simulink model "soc_range_doppler_fpga"  (R2025b)
settings: Solver=FixedStepDiscrete  StartTime=0.0  StopTime=inf  FixedStep=1/FPGAClkRate  RelTol=1e-3
values from neighbouring files (symbols this model uses):
  FPGAClkRate = Fs / SamplesPerClockCycle    (= 125000000)    [fmcw_run_test.m]    (also in soc_fmcw_init.m = 200000000)
  pulsePeriodSamples = ChirpSamples + 50    (= 1074)    [soc_range_doppler_system_param_init.m]    (also in soc_range_doppler_system_param_init_PDR_backup.m = 1952)
  pulseWidthSamples = 32    [soc_range_doppler_system_param_init.m]    (also in soc_range_doppler_system_param_init_PDR_backup.m)
  RngDimLen = ChirpSamples    (= 1024)    [soc_fmcw_init.m]    (also in soc_range_doppler_system_param_init.m; soc_range_doppler_system_param_init_PDR_backup.m)
  RxActiveSamples = ChirpSamples    (= 1024)    [soc_range_doppler_system_param_init.m]    (also in soc_range_doppler_system_param_init_PDR_backup.m)
  SamplesPerClockCycle = 2    [fmcw_run_test.m]    (also in soc_fmcw_init.m)
  TsFPGA = 1 / FPGAClkRate    (= 5e-09)    [soc_fmcw_init.m]
  txSignal = exp(1j * chirpPhase_short)    [soc_range_doppler_system_param_init.m]    (also in soc_range_doppler_system_param_init_PDR_backup.m = txSignalFullPeriod(1:pulseWidthSamples))
  VelDimLen = CPILength    (= 256)    [soc_fmcw_init.m]    (also in soc_range_doppler_system_param_init.m = 64; soc_range_doppler_system_param_init_PDR_backup.m = 64)
undefined symbols (not defined in the file or in its folder): NumBits1, NumBits2, TargetEmulator_MaxDelayLength, TargetEmulator_NCO_out_wl, TargetEmulator_NumChannels
libraries: simulink x9, socmemlib x8, hdlsllib x7, hwlogicconnlib x3, dsphdlsigops2 x1
(part 1 of 2)
settings Model: DataTypeOverride=Off  ModifiedByFormat=The MathWorks, Inc.  Creator=The MathWorks, Inc.  LastModifiedBy=The MathWorks, Inc.
settings SolverCC: AlgebraicLoopSolver=TrustRegion
settings DataIOCC: LimitDataPoints=on  SaveFormat=Array  SaveOutput=off  SaveTime=off  ReturnWorkspaceOutputs=off
settings OptimizationCC: BlockReduction=off  ConditionallyExecuteInputs=off  DefaultParameterBehavior=Inlined  ReuseModelBlockBuffer=off  LifeSpan=inf
settings DebuggingCC: AlgebraicLoopMsg=error  SolverPrmCheckMsg=warning  InheritedTsInSrcMsg=none  SingleTaskRateTransMsg=error  IntegerOverflowMsg=none  ParameterPrecisionLossMsg=none  UnconnectedInputMsg=warning  UnconnectedOutputMsg=warning  UnconnectedLineMsg=warning  AllowSymbolicDim=off  SFUnexpectedBacktrackingDiag=warning  SFNoUnconditionalDefaultTransitionDiag=warning  SFExecutionAtInitializationDiag=none  IntegerSaturationMsg=none  ArithmeticOperatorsInVariantConditions=warning
settings HardwareCC: ProdBitPerPointer=32.0  ProdBitPerSizeT=32.0  ProdBitPerPtrDiffT=32.0  ProdLargestAtomicFloat=None  ProdIntDivRoundTo=Undefined  ProdEndianess=Unspecified  ProdWordSize=32.0  ProdHWDeviceType=ASIC/FPGA->ASIC/FPGA  TargetBitPerPointer=64.0  TargetBitPerSizeT=64.0  TargetBitPerPtrDiffT=64.0  TargetLongLongMode=on  TargetIntDivRoundTo=Zero  TargetEndianess=LittleEndian  TargetWordSize=64.0  TargetHWDeviceType=Custom Processor->MATLAB Host Computer  ProdEqTarget=off
settings ModelReferenceCC: EnableRefExpFcnMdlSchedulingChecks=on  ModelReferenceNumInstancesAllowed=Single  PropagateSignalLabelsOutOfModel=off
settings SFSimCC: SimUseLocalCustomCode=off  CustomCodeUndefinedFunction=UseInterfaceOnly
settings RTWCC: RTWUseLocalCustomCode=off  GPUComputeCapability=3.5  DLArmComputeVersion=19.05
settings CodeAppCC: StateflowObjectComments=on
settings GRTTargetCC: TargetLangStandard=C89/C90 (ANSI)  SubcomponentCodeInterfacePackaging=Nonreusable function
settings ConfigComp: CovMetricSettings=dw  CovSaveCumulativeToWorkspaceVar=on  CovSaveSingleToWorkspaceVar=on  CovExternalEMLEnable=off  CovSFcnEnable=off
settings SimscapeCC: SimscapeNormalizeSystem=off

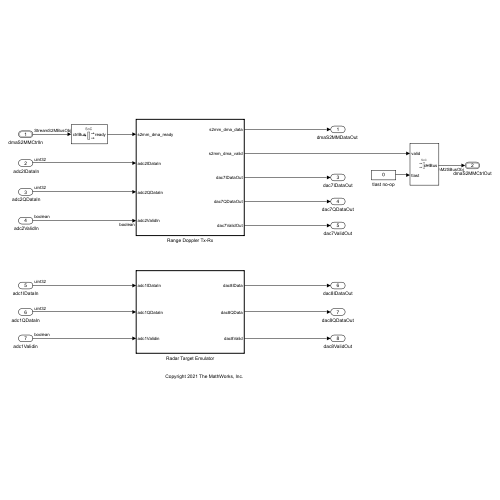
[thumbnail: Simulink's stored preview of the top-level diagram]
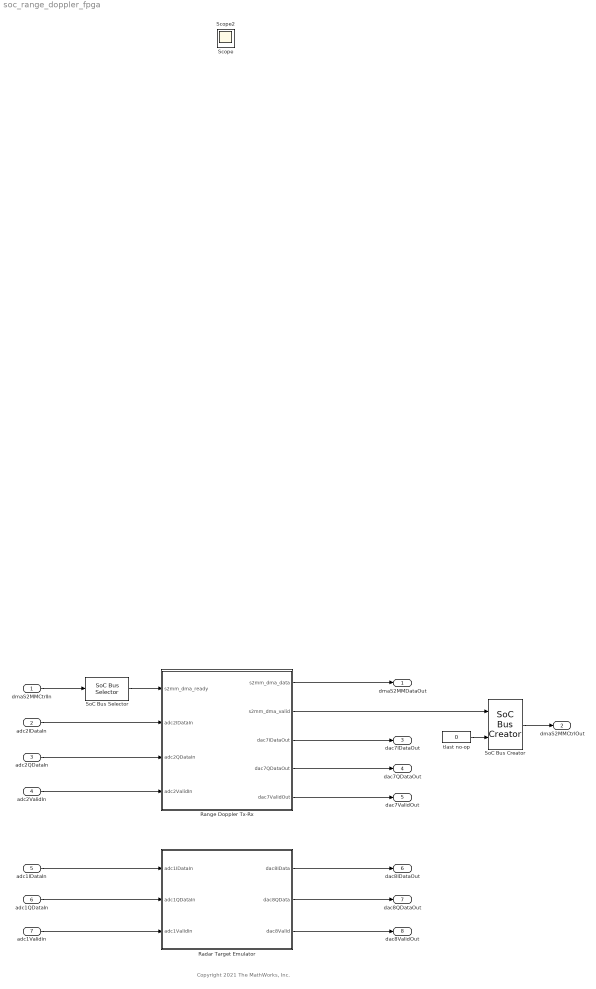
== system soc_range_doppler_fpga ==
  note: Copyright 2021 The MathWorks, Inc.
  dmaS2MMCtrlIn : Inport  OutDataTypeStr=Bus: StreamS2MBusObj  BusOutputAsStruct=on
  " adc2IDataIn" : Inport  Port=2  OutDataTypeStr=uint32  SampleTime=1/FPGAClkRate
  " adc2QDataIn" : Inport  Port=3  OutDataTypeStr=uint32  SampleTime=1/FPGAClkRate
  " adc2ValidIn" : Inport  Port=4  OutDataTypeStr=boolean  SampleTime=1/FPGAClkRate
  adc1IDataIn : Inport  Port=5  OutDataTypeStr=uint32
  adc1QDataIn : Inport  Port=6  OutDataTypeStr=uint32
  adc1Validin : Inport  Port=7  OutDataTypeStr=boolean
  Radar Target Emulator : Subsystem  TreatAsAtomicUnit=on
  Range Doppler Tx-Rx : Subsystem  TreatAsAtomicUnit=on
  SoC Bus Creator : hwlogicconnlib/SoC Bus Creator  Protocol=Data stream  ctrltype=Valid
  SoC Bus Selector : hwlogicconnlib/SoC Bus Selector  Protocol=Data stream  ctrltype=Ready
  tlast no-op : Constant  Value=0  OutDataTypeStr=boolean  SampleTime=-1
  "dmaS2MMDataOut " : Outport
  dmaS2MMCtrlOut : Outport  Port=2  OutDataTypeStr=Bus: StreamM2SBusObj  BusOutputAsStruct=on
  dac7IDataOut : Outport  Port=3
  dac7QDataOut : Outport  Port=4
  dac7ValidOut : Outport  Port=5
  dac8IDataOut : Outport  Port=6
  dac8QDataOut : Outport  Port=7
  dac8ValidOut : Outport  Port=8
  Scope : Scope
      settings: TimeSpan=1e-8*10  TimeUnits=Metric (based on Time Span)  ActiveDisplayYMinimum=-0.125  ActiveDisplayYMaximum=1.125
  Scope2 : Scope
      settings: ActiveDisplayYMinimum=-0.125  ActiveDisplayYMaximum=1.125
  wires:
  SoC Bus Creator/1 -> dmaS2MMCtrlOut/1
  tlast no-op/1 -> SoC Bus Creator/2
  Range Doppler Tx-Rx/2(s2mm_dma_valid) -> SoC Bus Creator/1
  SoC Bus Selector/1 -> Range Doppler Tx-Rx/1(s2mm_dma_ready)
  dmaS2MMCtrlIn/1 -> SoC Bus Selector/1
  Range Doppler Tx-Rx/1(s2mm_dma_data) -> "dmaS2MMDataOut "/1
  " adc2ValidIn"/1 -> Range Doppler Tx-Rx/4(adc2ValidIn)
  " adc2QDataIn"/1 -> Range Doppler Tx-Rx/3(adc2QDataIn)
  " adc2IDataIn"/1 -> Range Doppler Tx-Rx/2(adc2IDataIn)
  Radar Target Emulator/2(dac8QData) -> dac8QDataOut/1
  adc1IDataIn/1 -> Radar Target Emulator/1(adc1IDataIn)
  Radar Target Emulator/1(dac8IData) -> dac8IDataOut/1
  adc1Validin/1 -> Radar Target Emulator/3(adc1Validin)
  Radar Target Emulator/3(dac8Valid) -> dac8ValidOut/1
  adc1QDataIn/1 -> Radar Target Emulator/2(adc1QDataIn)
  Range Doppler Tx-Rx/3(dac7IDataOut) -> dac7IDataOut/1
  Range Doppler Tx-Rx/4(dac7QDataOut) -> dac7QDataOut/1
  Range Doppler Tx-Rx/5(dac7ValidOut) -> dac7ValidOut/1

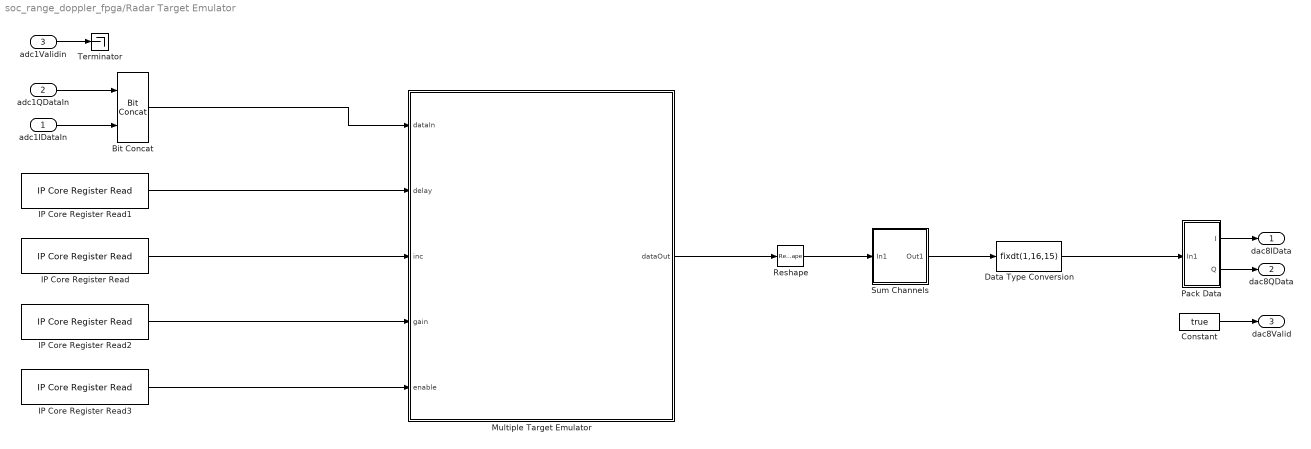
== system soc_range_doppler_fpga/Radar Target Emulator ==
  adc1IDataIn : Inport
  adc1QDataIn : Inport  Port=2
  adc1Validin : Inport  Port=3
  Bit Concat : hdlsllib/Logic and Bit Operations/Bit Concat  numInputs=2
  Constant : Constant  Value=true  SampleTime=-1
  Data Type Conversion : DataTypeConversion  OutDataTypeStr=fixdt(1,16,15)  SaturateOnIntegerOverflow=off  RndMeth=Floor
  IP Core Register Read : socmemlib/IP Core Register Read  RegisterName=Target_Emulator_Doppler_Inc  OutDataTypeStr=int32  OutputVectorSize=4  SampleTime=TsFPGA
  IP Core Register Read1 : socmemlib/IP Core Register Read  RegisterName=Target_Emulator_Range_Delay  OutDataTypeStr=uint32  OutputVectorSize=4  SampleTime=TsFPGA
  IP Core Register Read2 : socmemlib/IP Core Register Read  RegisterName=Target_Emulator_Gain  OutDataTypeStr=fixdt(1,18,17)  OutputVectorSize=4  SampleTime=TsFPGA
  IP Core Register Read3 : socmemlib/IP Core Register Read  RegisterName=Target_Emulator_Channel_Enable  OutDataTypeStr=boolean  OutputVectorSize=4  SampleTime=TsFPGA
  Multiple Target Emulator : Subsystem
  Pack Data : Subsystem
  Reshape : Reshape  OutputDimensionality=Customize  OutputDimensions=[SamplesPerClockCycle,TargetEmulator_NumChannels]
  Sum Channels : Subsystem
  Terminator : Terminator
  dac8IData : Outport
  dac8QData : Outport  Port=2
  dac8Valid : Outport  Port=3
  wires:
  adc1Validin/1 -> Terminator/1
  Constant/1 -> dac8Valid/1
  adc1IDataIn/1 -> Bit Concat/2
  adc1QDataIn/1 -> Bit Concat/1
  Pack Data/1(I) -> dac8IData/1
  Pack Data/2(Q) -> dac8QData/1
  Bit Concat/1 -> Multiple Target Emulator/1(dataIn)
  IP Core Register Read1/1 -> Multiple Target Emulator/2(delay)
  IP Core Register Read/1 -> Multiple Target Emulator/3(inc)
  IP Core Register Read2/1 -> Multiple Target Emulator/4(gain)
  Multiple Target Emulator/1(dataOut) -> Reshape/1
  Data Type Conversion/1 -> Pack Data/1(In1)
  IP Core Register Read3/1 -> Multiple Target Emulator/5(enable)
  Reshape/1 -> Sum Channels/1(In1)
  Sum Channels/1(Out1) -> Data Type Conversion/1

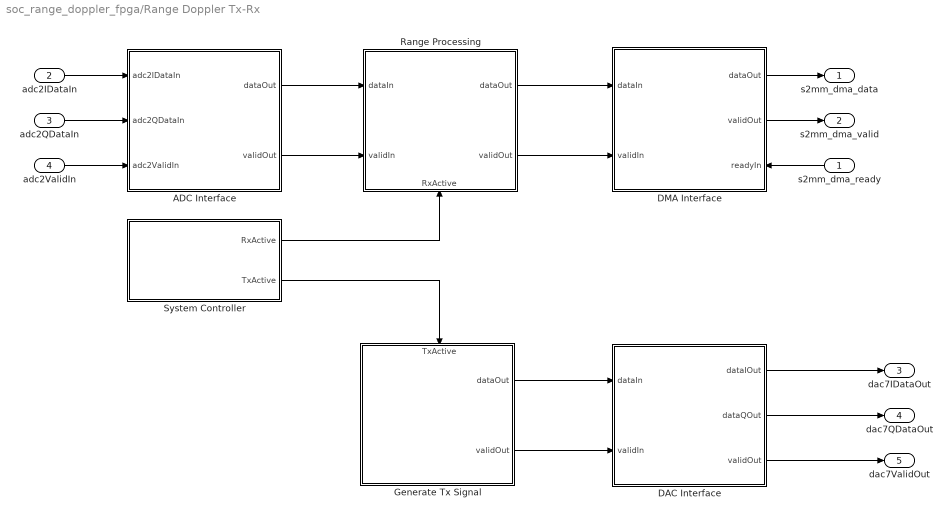
== system soc_range_doppler_fpga/Range Doppler Tx-Rx ==
  s2mm_dma_ready : Inport
  adc2IDataIn : Inport  Port=2  SampleTime=1/FPGAClkRate
  adc2QDataIn : Inport  Port=3  SampleTime=1/FPGAClkRate
  adc2ValidIn : Inport  Port=4  OutDataTypeStr=boolean  SampleTime=1/FPGAClkRate
  ADC Interface : Subsystem
  DAC Interface : Subsystem
  DMA Interface : Subsystem
      settings: PortSchema="{\"entries\":[{\"content\":{\"sides\":[{\"content\":{\"connectorIds\":[\"In1\",\"In2\"]},\"type\":\"ConnectorPlacement.EquallySpacedRectSide\",\"uuid\":\"5e6ee6ef-653d-4c22-91ec-0e4d08fe2bda\"},{\"content\":{\"connectorIds\":[\"Out1\",\"Out2\",\"In3\"],\"side\":\"RIGHT\"},\"type\":\"ConnectorPlacement.EquallySpacedRectSide\",\"uuid\":\"cc17ec3f-1a41-4b37-b05d-9322698b0460\"},{\"content\":{\"connectorIds\":[],\"side\":\"TOP\"},\"type\":\"ConnectorPlacement.EquallySpacedRectSide\",\"uuid\":\"ad44321b-ea67-4558-a5e3-5d4593ef958c\"},{\"content\":{\"connectorIds\":[],\"side\":\"HIDDEN\"},\"type\":\"ConnectorPlacement.EquallySpacedRectSide\",\"uuid\":\"4d1513b6-023e-4107-a61f-cebca5303f4a\"}]},\"type\":\"ConnectorPlacement.EquallySpacedConnector\",\"uuid\":\"368f7437-0e21-4f0c-b817-b9c98445f229\"}],\"packageUris\":[\"http://schema.mathworks.com/mf0/Connector/R2020b\"],\"version\":\"1.0\"}"
  Generate Tx Signal : Subsystem
      settings: PortSchema="{\"entries\":[{\"content\":{\"sides\":[{\"content\":{\"connectorIds\":[]},\"type\":\"ConnectorPlacement.EquallySpacedRectSide\",\"uuid\":\"7c0c8442-b2b4-479b-a8c5-9f379b7e9b02\"},{\"content\":{\"connectorIds\":[\"Out1\",\"Out2\"],\"side\":\"RIGHT\"},\"type\":\"ConnectorPlacement.EquallySpacedRectSide\",\"uuid\":\"78e009c0-26e1-4601-bc88-d3b747828f60\"},{\"content\":{\"connectorIds\":[\"In1\"],\"side\":\"TOP\"},\"type\":\"ConnectorPlacement.EquallySpacedRectSide\",\"uuid\":\"f420d1c4-59cf-4bc3-a158-4cd82eb58765\"},{\"content\":{\"connectorIds\":[],\"side\":\"BOTTOM\"},\"type\":\"ConnectorPlacement.EquallySpacedRectSide\",\"uuid\":\"c7f1fd46-69ec-4218-a957-5990432ef52d\"},{\"content\":{\"connectorIds\":[],\"side\":\"HIDDEN\"},\"type\":\"ConnectorPlacement.EquallySpacedRectSide\",\"uuid\":\"a6a12a6f-fd1c-4a75-bd3d-72d2093a42d1\"}]},\"type\":\"ConnectorPlacement.EquallySpacedConnector\",\"uuid\":\"fef31356-b6d9-440d-aa7f-68d9fbecd58b\"}],\"packageUris\":[\"http://schema.mathworks.com/mf0/Connector/R2020b\"],\"version\":\"1.0\"}"
  Range Processing : Subsystem
      settings: PortSchema="{\"entries\":[{\"content\":{\"sides\":[{\"content\":{\"connectorIds\":[\"In1\",\"In2\"]},\"type\":\"ConnectorPlacement.EquallySpacedRectSide\",\"uuid\":\"39bc8e28-b2f1-4549-a29c-f4f4cd813fa8\"},{\"content\":{\"connectorIds\":[\"Out1\",\"Out2\"],\"side\":\"RIGHT\"},\"type\":\"ConnectorPlacement.EquallySpacedRectSide\",\"uuid\":\"b450daac-133f-42c0-b4eb-be8f21a05aa1\"},{\"content\":{\"connectorIds\":[],\"side\":\"TOP\"},\"type\":\"ConnectorPlacement.EquallySpacedRectSide\",\"uuid\":\"67fab3c9-6d2a-4d44-89b3-69577d01f951\"},{\"content\":{\"connectorIds\":[\"In3\"],\"side\":\"BOTTOM\"},\"type\":\"ConnectorPlacement.EquallySpacedRectSide\",\"uuid\":\"f598741e-2794-4676-b4d9-8ec658bb222d\"},{\"content\":{\"connectorIds\":[],\"side\":\"HIDDEN\"},\"type\":\"ConnectorPlacement.EquallySpacedRectSide\",\"uuid\":\"bbc24f9c-adbc-4398-b2a6-1edaf7ae5a6a\"}]},\"type\":\"ConnectorPlacement.EquallySpacedConnector\",\"uuid\":\"0f1d461d-e89e-4ae5-bc4e-aa440f4196de\"}],\"packageUris\":[\"http://schema.mathworks.com/mf0/Connector/R2020b\"],\"version\":\"1.0\"}"
  System Controller : Subsystem
  s2mm_dma_data : Outport
  s2mm_dma_valid : Outport  Port=2
  dac7IDataOut : Outport  Port=3
  dac7QDataOut : Outport  Port=4
  dac7ValidOut : Outport  Port=5
  wires:
  DMA Interface/1(dataOut) -> s2mm_dma_data/1
  s2mm_dma_ready/1 -> DMA Interface/3(readyIn)
  DMA Interface/2(validOut) -> s2mm_dma_valid/1
  DAC Interface/1(dataIOut) -> dac7IDataOut/1
  DAC Interface/2(dataQOut) -> dac7QDataOut/1
  DAC Interface/3(validOut) -> dac7ValidOut/1
  System Controller/2(TxActive) -> Generate Tx Signal/1(TxActive)
  Range Processing/1(dataOut) -> DMA Interface/1(dataIn)
  System Controller/1(RxActive) -> Range Processing/3(RxActive)
  Generate Tx Signal/1(dataOut) -> DAC Interface/1(dataIn)
  Generate Tx Signal/2(validOut) -> DAC Interface/2(validIn)
  Range Processing/2(validOut) -> DMA Interface/2(validIn)
  ADC Interface/1(dataOut) -> Range Processing/1(dataIn)
  ADC Interface/2(validOut) -> Range Processing/2(validIn)
  adc2IDataIn/1 -> ADC Interface/1(adc2IDataIn)
  adc2QDataIn/1 -> ADC Interface/2(adc2QDataIn)
  adc2ValidIn/1 -> ADC Interface/3(adc2ValidIn)

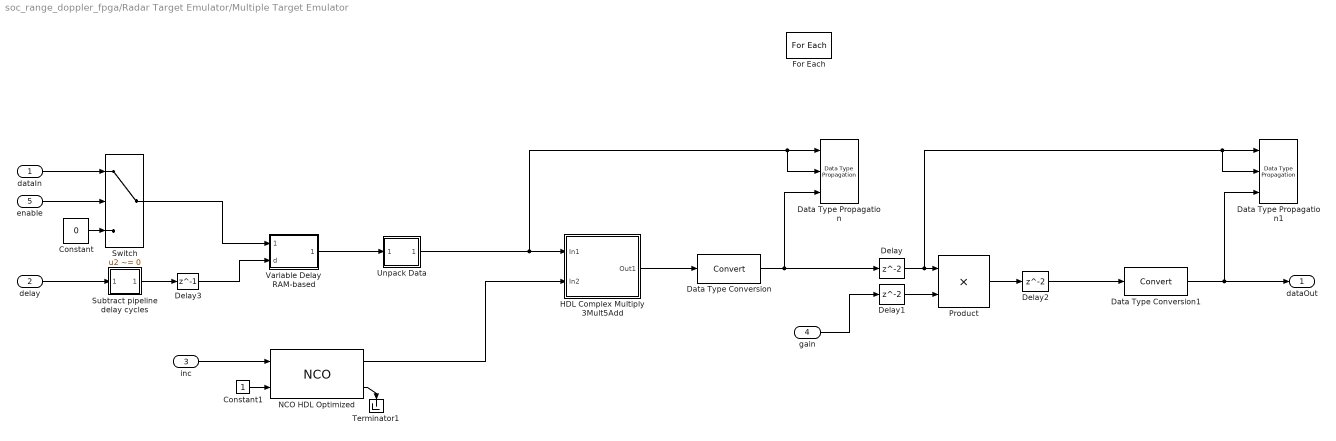
== system soc_range_doppler_fpga/Radar Target Emulator/Multiple Target Emulator ==
  dataIn : Inport
  delay : Inport  Port=2  Partition=on  PartitionDimension=1  PartitionWidth=1  PartitionOffset=0
  inc : Inport  Port=3  Partition=on  PartitionDimension=1  PartitionWidth=1  PartitionOffset=0
  gain : Inport  Port=4  Partition=on  PartitionDimension=1  PartitionWidth=1  PartitionOffset=0
  enable : Inport  Port=5  Partition=on  PartitionDimension=1  PartitionWidth=1  PartitionOffset=0
  Constant : Constant  Value=0  OutDataTypeStr=Inherit: Inherit via back propagation  SampleTime=-1
  Constant1 : Constant  OutDataTypeStr=boolean  SampleTime=-1
  Data Type Propagation : simulink/Signal Attributes/Data Type Propagation  PropDataTypeMode=Specify via dialog  PropDataType=fixdt(1, 24)  IfRefDouble=double  IfRefSingle=single  IsSigned=IsSigned1 or IsSigned2  NumBitsBase=max([NumBits1 NumBits2])  NumBitsMult=1  NumBitsAdd=0  NumBitsAllowFinal=1:24  PropScaling=2^-10  ValuesUsedBestPrec=[5 -7]  SlopeBase=PosRange1  SlopeMult=1  SlopeAdd=0  BiasBase=Bias1  BiasMult=1  BiasAdd=0
  Data Type Propagation1 : simulink/Signal Attributes/Data Type Propagation  PropDataTypeMode=Specify via dialog  PropDataType=fixdt(1, 16)  IfRefDouble=double  IfRefSingle=single  IsSigned=IsSigned1 or IsSigned2  NumBitsBase=max([NumBits1 NumBits2])  NumBitsMult=1  NumBitsAdd=0  NumBitsAllowFinal=1:24  PropScaling=2^-10  ValuesUsedBestPrec=[5 -7]  SlopeBase=PosRange1  SlopeMult=1  SlopeAdd=0  BiasBase=Bias1  BiasMult=1  BiasAdd=0
  Data Type Conversion : DataTypeConversion  SaturateOnIntegerOverflow=off  RndMeth=Floor
  Data Type Conversion1 : DataTypeConversion  SaturateOnIntegerOverflow=off  RndMeth=Floor
  Delay : Delay
  Delay1 : Delay
  Delay2 : Delay
  Delay3 : Delay  DelayLength=1
  For Each : ForEach  DisableCoverage=on
  HDL Complex Multiply 3Mult5Add : Subsystem  mask(HDL Complex Multiplier (3 Multiply, 5 Add)){D1=2, D2=1, D3=1, D4=1, D5=1}
      mask help:
      | Xilinx devices:
      | - Set D1 = 1 or 2 to trade off speed & FF resources
      | - Set D2-D5 = 1 to fully leverage DSP48 pipelines
      | - Use sync reset
      |
      | Intel FPGAs:
      | - Set D1 = 1 or 2 depending on device family
      | - Set D5 = 1; D2, D3, D4 = 0
      | - Use async reset
      mask init:
      | delay = D1+D2+D3+D4+D5;
  NCO HDL Optimized : dsphdlsigops2/NCO  PhaseIncrementSource=Input port  PhaseIncrement=100  PhaseOffsetSource=Property  PhaseOffset=0  DitherSource=Property  NumDitherBits=TargetEmulator_NCO_dither_wl  SamplesPerFrame=1  LUTCompress=on  ResetAction=off  Waveform=Complex exponential  PhasePort=off  SimulateUsing=Code generation  AccumulatorWL=TargetEmulator_NCO_accum_wl  PhaseQuantization=on  NumQuantizerAccumulatorBits=TargetEmulator_NCO_quantizer_wl  OutputDataType=Binary point scaling  OutputWL=TargetEmulator_NCO_out_wl  OutputFL=TargetEmulator_NCO_out_wl-1
  Product : Product
  Subtract pipeline delay cycles : Subsystem  mask{C=12 + nextpow2(TargetEmulator_NumChannels)}
      mask prompts: C "Constant"
      mask init:
      | dt = fixdt(1,nextpow2(C)+1,0);
      mask Display:
      | Cstr = get_param(gcb,'C');
      | 
      | fprintf('u-%s',Cstr);
  Switch : Switch  Criteria=u2 ~= 0  SaturateOnIntegerOverflow=off  InputSameDT=off
  Terminator1 : Terminator
  Unpack Data : Subsystem
  Variable Delay RAM-based : Subsystem  mask(RAM-based variable delay){MAX_DELAY=TargetEmulator_MaxDelayLength}
      mask prompts: MAX_DELAY "Maximum delay length:"
      mask TypeOptions MAX_DELAY: Variable Delay RAM Based/MAX_DELAY
      mask Display:
      | text(0.5,0.5,'z^{-d-1}','horizontalAlignment','center',...
      |     'verticalAlignment','middle','texmode','on');
      | 
      | port_label('input',1,'u');
      | port_label('input',2,'d');
  dataOut : Outport  ConcatenationDimension=1
  wires:
  NCO HDL Optimized/2 -> Terminator1/1
  Delay2/1 -> Data Type Conversion1/1
  Constant1/1 -> NCO HDL Optimized/2
  Delay3/1 -> Variable Delay RAM-based/2(d)
  Unpack Data/1(Out1) -> Data Type Propagation/2, Data Type Propagation/1, HDL Complex Multiply 3Mult5Add/1(In1)
  inc/1 -> NCO HDL Optimized/1
  Product/1 -> Delay2/1
  Variable Delay RAM-based/1(dataOut) -> Unpack Data/1(In1)
  Data Type Conversion/1 -> Data Type Propagation/3, Delay/1
  Subtract pipeline delay cycles/1(Out1) -> Delay3/1
  HDL Complex Multiply 3Mult5Add/1(Out1) -> Data Type Conversion/1
  NCO HDL Optimized/1 -> HDL Complex Multiply 3Mult5Add/2(In2)
  Data Type Conversion1/1 -> dataOut/1, Data Type Propagation1/3
  Delay/1 -> Data Type Propagation1/2, Data Type Propagation1/1, Product/1
  Delay1/1 -> Product/2
  delay/1 -> Subtract pipeline delay cycles/1(In1)
  gain/1 -> Delay1/1
  enable/1 -> Switch/2
  Switch/1 -> Variable Delay RAM-based/1(dataIn)
  dataIn/1 -> Switch/1
  Constant/1 -> Switch/3

== system soc_range_doppler_fpga/Radar Target Emulator/Pack Data ==
  In1 : Inport
  Complex to Real-Imag : ComplexToRealImag
  Pack Vector : Subsystem  mask(Pack Vector){}
      mask help:
      | Convert vector to packed word.
      |
      | The first vector element is placed in the LSB, and the last vector element is placed in the MSB.
      mask Display: fprintf('Pack\nVector');
  Pack Vector1 : Subsystem  mask(Pack Vector){}
      mask help:
      | Convert vector to packed word.
      |
      | The first vector element is placed in the LSB, and the last vector element is placed in the MSB.
      mask Display: fprintf('Pack\nVector');
  I : Outport
  Q : Outport  Port=2
  wires:
  In1/1 -> Complex to Real-Imag/1
  Complex to Real-Imag/1 -> Pack Vector/1(u)
  Complex to Real-Imag/2 -> Pack Vector1/1(u)
  Pack Vector/1(y) -> I/1
  Pack Vector1/1(y) -> Q/1

== system soc_range_doppler_fpga/Radar Target Emulator/Sum Channels ==
  In1 : Inport
  Delay : Delay  DelayLength=nextpow2(TargetEmulator_NumChannels)
  Sum of Elements : Sum  Inputs=+  CollapseMode=Specified dimension  CollapseDim=2
  Out1 : Outport
  wires:
  In1/1 -> Sum of Elements/1
  Sum of Elements/1 -> Delay/1
  Delay/1 -> Out1/1

== system soc_range_doppler_fpga/Range Doppler Tx-Rx/ADC Interface ==
  adc2IDataIn : Inport  SampleTime=1/FPGAClkRate
  adc2QDataIn : Inport  Port=2  SampleTime=1/FPGAClkRate
  adc2ValidIn : Inport  Port=3  OutDataTypeStr=boolean  SampleTime=1/FPGAClkRate
  Data Type Conversion2 : DataTypeConversion  OutDataTypeStr=inputDT  SaturateOnIntegerOverflow=off  RndMeth=Floor
  Real-Imag to Complex : RealImagToComplex
  Unpack Vector I : Subsystem  mask(Convert packed word to vector.){datatype=fixdt(1,16,15), VectorLength=SamplesPerClockCycle}
      mask prompts: datatype "Output datatype:"; VectorLength "Vector length:"
      mask help: Input word has the first vector element in the LSB and the last element in the MSB.
      mask init:
      | OutputWordLength = numerictype(datatype).WordLength;
      | 
      | Simulink.suppressDiagnostic(gcbh,...
      |  'SimulinkFixedPoint:util:Overflowoccurred');
      mask Display: fprintf('Unpack\nVector');
  Unpack Vector Q : Subsystem  mask(Convert packed word to vector.){datatype=fixdt(1,16,15), VectorLength=SamplesPerClockCycle}
      mask prompts: datatype "Output datatype:"; VectorLength "Vector length:"
      mask help: Input word has the first vector element in the LSB and the last element in the MSB.
      mask init:
      | OutputWordLength = numerictype(datatype).WordLength;
      | 
      | Simulink.suppressDiagnostic(gcbh,...
      |  'SimulinkFixedPoint:util:Overflowoccurred');
      mask Display: fprintf('Unpack\nVector');
  dataOut : Outport
  validOut : Outport  Port=2
  wires:
  adc2IDataIn/1 -> Unpack Vector I/1(In1)
  Real-Imag to Complex/1 -> Data Type Conversion2/1
  Unpack Vector Q/1(Out1) -> Real-Imag to Complex/2
  Unpack Vector I/1(Out1) -> Real-Imag to Complex/1
  Data Type Conversion2/1 -> dataOut/1
  adc2ValidIn/1 -> validOut/1
  adc2QDataIn/1 -> Unpack Vector Q/1(In1)

== system soc_range_doppler_fpga/Range Doppler Tx-Rx/DAC Interface ==
  dataIn : Inport
  validIn : Inport  Port=2
  Complex to Real-Imag : ComplexToRealImag
  Pack Vector I : Subsystem  mask(Pack Vector){}
      mask help:
      | Convert vector to packed word.
      |
      | The first vector element is placed in the LSB, and the last vector element is placed in the MSB.
      mask Display: fprintf('Pack\nVector');
  Pack Vector Q : Subsystem  mask(Pack Vector){}
      mask help:
      | Convert vector to packed word.
      |
      | The first vector element is placed in the LSB, and the last vector element is placed in the MSB.
      mask Display: fprintf('Pack\nVector');
  dataIOut : Outport
  dataQOut : Outport  Port=2
  validOut : Outport  Port=3
  wires:
  Complex to Real-Imag/1 -> Pack Vector I/1(u)
  Complex to Real-Imag/2 -> Pack Vector Q/1(u)
  Pack Vector I/1(y) -> dataIOut/1
  Pack Vector Q/1(y) -> dataQOut/1
  dataIn/1 -> Complex to Real-Imag/1
  validIn/1 -> validOut/1

== system soc_range_doppler_fpga/Range Doppler Tx-Rx/DMA Interface ==
  dataIn : Inport
  validIn : Inport  Port=2
  readyIn : Inport  Port=3
  Pack Complex Vector : Subsystem  mask(Pack Complex Vector){}
      mask help:
      | Convert complex vector to packed word.
      |
      | Real and imaginary components are interleaved, with real component starting in LSB position.
      |
      | The first vector element is placed in the LSB, and the last vector element is placed in the MSB.
      mask Display: fprintf('Pack\nComplex\nVector');
  Stream FIFO : hwlogicconnlib/Stream FIFO  FIFO_DEPTH=1024  AFULL_THRESH=1023
  Terminator : Terminator
  dataOut : Outport
  validOut : Outport  Port=2
  wires:
  dataIn/1 -> Pack Complex Vector/1(u)
  Stream FIFO/1 -> dataOut/1
  Stream FIFO/2 -> validOut/1
  readyIn/1 -> Stream FIFO/3
  Pack Complex Vector/1(y) -> Stream FIFO/1
  validIn/1 -> Stream FIFO/2
  Stream FIFO/3 -> Terminator/1

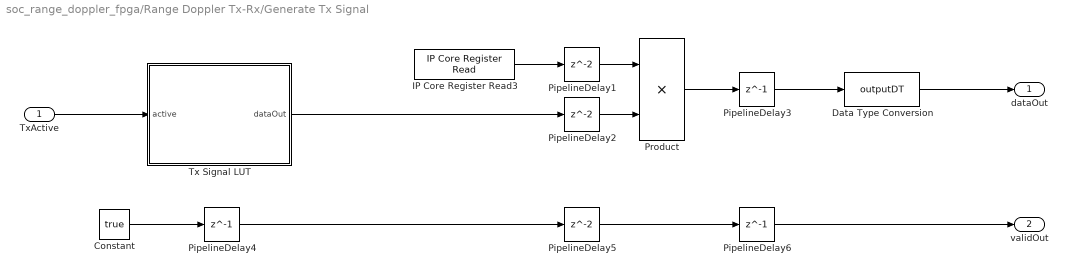
== system soc_range_doppler_fpga/Range Doppler Tx-Rx/Generate Tx Signal ==
  TxActive : Inport
  Constant : Constant  Value=true  SampleTime=-1
  Data Type Conversion : DataTypeConversion  OutDataTypeStr=outputDT  SaturateOnIntegerOverflow=off  RndMeth=Floor
  IP Core Register Read3 : socmemlib/IP Core Register Read  RegisterName=Tx_Gain  OutDataTypeStr=fixdt(1,18,16)  OutputVectorSize=1  SampleTime=TsFPGA
  PipelineDelay1 : Delay
  PipelineDelay2 : Delay
  PipelineDelay3 : Delay  DelayLength=1
  PipelineDelay4 : Delay  DelayLength=1
  PipelineDelay5 : Delay
  PipelineDelay6 : Delay  DelayLength=1
  Product : Product
  Tx Signal LUT : Subsystem
  dataOut : Outport
  validOut : Outport  Port=2
  wires:
  Product/1 -> PipelineDelay3/1
  PipelineDelay3/1 -> Data Type Conversion/1
  PipelineDelay2/1 -> Product/2
  PipelineDelay1/1 -> Product/1
  IP Core Register Read3/1 -> PipelineDelay1/1
  Tx Signal LUT/1(dataOut) -> PipelineDelay2/1
  TxActive/1 -> Tx Signal LUT/1(active)
  Data Type Conversion/1 -> dataOut/1
  Constant/1 -> PipelineDelay4/1
  PipelineDelay4/1 -> PipelineDelay5/1
  PipelineDelay5/1 -> PipelineDelay6/1
  PipelineDelay6/1 -> validOut/1

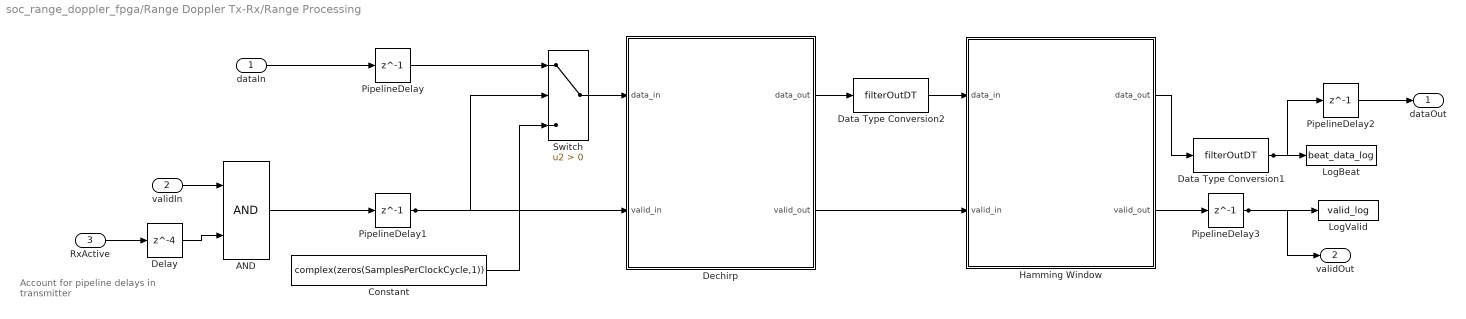
== system soc_range_doppler_fpga/Range Doppler Tx-Rx/Range Processing ==
  note: Account for pipeline
      | delays in transmitter
  dataIn : Inport
  validIn : Inport  Port=2
  RxActive : Inport  Port=3
  AND : Logic  IconShape=distinctive  AllPortsSameDT=off  OutDataTypeStr=boolean
  Constant : Constant  Value=complex(zeros(SamplesPerClockCycle,1))  OutDataTypeStr=inputDT  SampleTime=-1
  Data Type Conversion1 : DataTypeConversion  OutDataTypeStr=filterOutDT  SaturateOnIntegerOverflow=off  RndMeth=Floor
  Data Type Conversion2 : DataTypeConversion  OutDataTypeStr=filterOutDT  SaturateOnIntegerOverflow=off  RndMeth=Floor
  Dechirp : Subsystem
  Delay : Delay  DelayLength=4
  Hamming Window : Subsystem
  LogBeat : ToWorkspace  VariableName=beat_data_log  SaveFormat=Timeseries  SampleTime=-1
  LogValid : ToWorkspace  VariableName=valid_log  SaveFormat=Timeseries  SampleTime=-1
  PipelineDelay{,1..3} (4 alike) : Delay  DelayLength=1
  Switch : Switch  Criteria=u2 > Threshold  SaturateOnIntegerOverflow=off  InputSameDT=off
  dataOut : Outport
  validOut : Outport  Port=2
  wires:
  validIn/1 -> AND/1
  RxActive/1 -> Delay/1
  Constant/1 -> Switch/3
  PipelineDelay/1 -> Switch/1
  Delay/1 -> AND/2
  dataIn/1 -> PipelineDelay/1
  AND/1 -> PipelineDelay1/1
  PipelineDelay1/1 -> Dechirp/2(valid_in), Switch/2
  PipelineDelay2/1 -> dataOut/1
  Switch/1 -> Dechirp/1(data_in)
  Dechirp/1(data_out) -> Data Type Conversion2/1
  Dechirp/2(valid_out) -> Hamming Window/2(valid_in)
  Data Type Conversion2/1 -> Hamming Window/1(data_in)
  Hamming Window/1(data_out) -> Data Type Conversion1/1
  Hamming Window/2(valid_out) -> PipelineDelay3/1
  Data Type Conversion1/1 -> PipelineDelay2/1, LogBeat/1
  PipelineDelay3/1 -> validOut/1, LogValid/1

== system soc_range_doppler_fpga/Range Doppler Tx-Rx/System Controller ==
  IP Core Register Read : socmemlib/IP Core Register Read  RegisterName=CPI_Start  OutDataTypeStr=boolean  OutputVectorSize=1  SampleTime=TsFPGA
  IP Core Register Read1 : socmemlib/IP Core Register Read  RegisterName=CPI_Length  OutDataTypeStr=uint32  OutputVectorSize=1  SampleTime=TsFPGA
  IP Core Register Read2 : socmemlib/IP Core Register Read  RegisterName=Rx_Delay_Cycles  OutDataTypeStr=uint32  OutputVectorSize=1  SampleTime=TsFPGA
  System Controller Fcn : MATLAB Function  TreatAsAtomicUnit=on
  RxActive : Outport
  TxActive : Outport  Port=2
  wires:
  IP Core Register Read2/1 -> System Controller Fcn/3(rx_delay_cycles)
  IP Core Register Read1/1 -> System Controller Fcn/2(cpi_length)
  IP Core Register Read/1 -> System Controller Fcn/1(cpi_start)
  System Controller Fcn/1(tx_active) -> TxActive/1
  System Controller Fcn/2(rx_active) -> RxActive/1

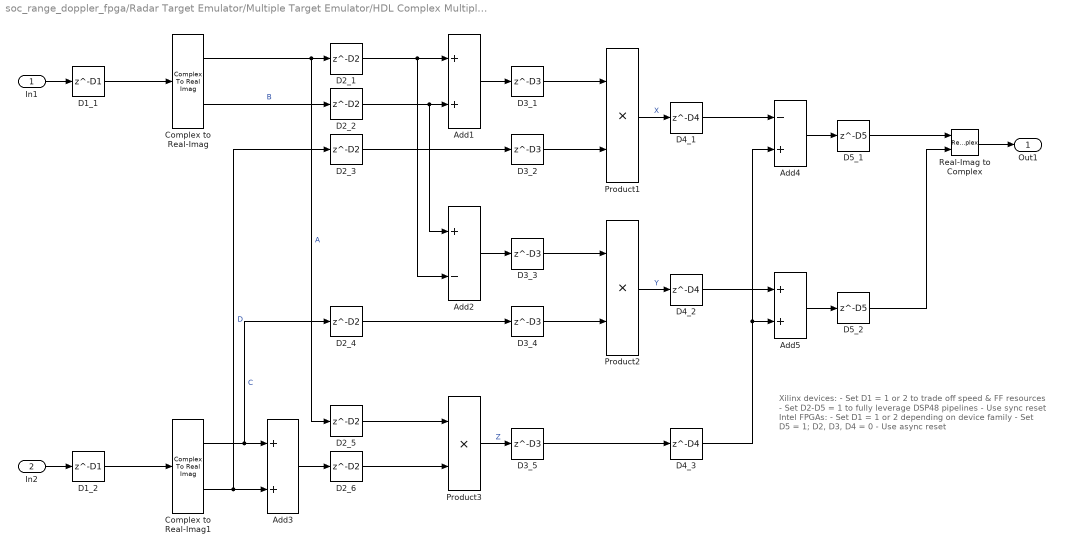
== system soc_range_doppler_fpga/Radar Target Emulator/Multiple Target Emulator/HDL Complex Multiply 3Mult5Add ==
  note: Xilinx devices:
      | - Set D1 = 1 or 2 to trade off speed & FF resources
      | - Set D2-D5 = 1 to fully leverage DSP48 pipelines
      | - Use sync reset
      |
      | Intel FPGAs:
      | - Set D1 = 1 or 2 depending on device family
      | - Set D5 = 1; D2, D3, D4 = 0
      | - Use async reset
  In1 : Inport
  In2 : Inport  Port=2
  Add1 : Sum
  Add2 : Sum  Inputs=+-
  Add3 : Sum
  Add4 : Sum  Inputs=-+
  Add5 : Sum
  Complex to Real-Imag : ComplexToRealImag
  Complex to Real-Imag1 : ComplexToRealImag
  D1_1 : Delay  DelayLength=D1
  D1_2 : Delay  DelayLength=D1
  D2_{1..6} (6 alike) : Delay  DelayLength=D2
  D3_{1..5} (5 alike) : Delay  DelayLength=D3
  D4_1 : Delay  DelayLength=D4
  D4_2 : Delay  DelayLength=D4
  D4_3 : Delay  DelayLength=D4
  D5_1 : Delay  DelayLength=D5
  D5_2 : Delay  DelayLength=D5
  Product1 : Product
  Product2 : Product
  Product3 : Product
  Real-Imag to Complex : RealImagToComplex
  Out1 : Outport  VectorParamsAs1DForOutWhenUnconnected=off
  wires:
  D1_2/1 -> Complex to Real-Imag1/1
  D1_1/1 -> Complex to Real-Imag/1
  In1/1 -> D1_1/1
  D2_1/1 -> Add1/1, Add2/2
  D2_2/1 -> Add2/1, Add1/2
  D2_5/1 -> Product3/1
  D2_3/1 -> D3_2/1
  D2_4/1 -> D3_4/1
  D3_2/1 -> Product1/2
  D3_4/1 -> Product2/2
  D4_3/1 -> Add5/2, Add4/2
  D3_3/1 -> Product2/1
  D2_6/1 -> Product3/2
  D3_1/1 -> Product1/1
  Complex to Real-Imag/2 -> D2_2/1  "B"
  Complex to Real-Imag/1 -> D2_1/1, D2_5/1  "A"
  Add2/1 -> D3_3/1
  Add3/1 -> D2_6/1
  Add1/1 -> D3_1/1
  D3_5/1 -> D4_3/1
  D4_2/1 -> Add5/1
  D4_1/1 -> Add4/1
  D5_2/1 -> Real-Imag to Complex/2
  D5_1/1 -> Real-Imag to Complex/1
  Add5/1 -> D5_2/1
  Add4/1 -> D5_1/1
  Product3/1 -> D3_5/1  "Z"
  Product2/1 -> D4_2/1  "Y"
  Product1/1 -> D4_1/1  "X"
  Complex to Real-Imag1/2 -> D2_3/1, Add3/2  "D"
  Complex to Real-Imag1/1 -> D2_4/1, Add3/1  "C"
  In2/1 -> D1_2/1
  Real-Imag to Complex/1 -> Out1/1

== system soc_range_doppler_fpga/Radar Target Emulator/Multiple Target Emulator/Subtract pipeline delay cycles ==
  In1 : Inport
  Constant : Constant  Value=C  OutDataTypeStr=dt  SampleTime=-1
  Subtract : Sum  Inputs=+-  OutDataTypeStr=Inherit: Same as accumulator
  Out1 : Outport
  wires:
  Constant/1 -> Subtract/2
  Subtract/1 -> Out1/1
  In1/1 -> Subtract/1

== system soc_range_doppler_fpga/Radar Target Emulator/Multiple Target Emulator/Unpack Data ==
  In1 : Inport
  Extract Bits : simulink/Logic and Bit Operations/Extract Bits  bitsToExtract=Lower half  numBits=8  bitIdxRange=[0 7]  outScalingMode=Treat bit field as an integer
  Extract Bits1 : simulink/Logic and Bit Operations/Extract Bits  bitsToExtract=Upper half  numBits=8  bitIdxRange=[0 7]  outScalingMode=Treat bit field as an integer
  Real-Imag to Complex : RealImagToComplex
  Unpack Vector : Subsystem  mask(Convert packed word to vector.){datatype=fixdt(1,16,15), VectorLength=SamplesPerClockCycle}
      mask prompts: datatype "Output datatype:"; VectorLength "Vector length:"
      mask help: Input word has the first vector element in the LSB and the last element in the MSB.
      mask init:
      | OutputWordLength = numerictype(datatype).WordLength;
      | 
      | Simulink.suppressDiagnostic(gcbh,...
      |  'SimulinkFixedPoint:util:Overflowoccurred');
      mask Display: fprintf('Unpack\nVector');
  Unpack Vector1 : Subsystem  mask(Convert packed word to vector.){datatype=fixdt(1,16,15), VectorLength=SamplesPerClockCycle}
      mask prompts: datatype "Output datatype:"; VectorLength "Vector length:"
      mask help: Input word has the first vector element in the LSB and the last element in the MSB.
      mask init:
      | OutputWordLength = numerictype(datatype).WordLength;
      | 
      | Simulink.suppressDiagnostic(gcbh,...
      |  'SimulinkFixedPoint:util:Overflowoccurred');
      mask Display: fprintf('Unpack\nVector');
  Out1 : Outport
  wires:
  In1/1 -> Extract Bits1/1, Extract Bits/1
  Extract Bits1/1 -> Unpack Vector1/1(In1)
  Extract Bits/1 -> Unpack Vector/1(In1)
  Unpack Vector/1(Out1) -> Real-Imag to Complex/1
  Unpack Vector1/1(Out1) -> Real-Imag to Complex/2
  Real-Imag to Complex/1 -> Out1/1

== system soc_range_doppler_fpga/Radar Target Emulator/Multiple Target Emulator/Variable Delay RAM-based ==
  dataIn : Inport
  d : Inport  Port=2
  Constant : Constant  Value=true  SampleTime=-1
  Terminator : Terminator
  Variable Delay RAM Based : Subsystem  mask{MAX_DELAY=MAX_DELAY}
      mask prompts: MAX_DELAY "Maximum delay length:"
      mask init:
      | ADDR_WIDTH = nextpow2(MAX_DELAY);
      | ADDR_DT = fixdt(0,ADDR_WIDTH,0);
      | IDX_DT = fixdt(1,ADDR_WIDTH+2,0);
      mask Display:
      | text(0.42, 0.5, 'Z');
      | text(0.47, 0.55, '-d-1');
  dataOut : Outport
  wires:
  Constant/1 -> Variable Delay RAM Based/2(validIn)
  Variable Delay RAM Based/2(validOut) -> Terminator/1
  dataIn/1 -> Variable Delay RAM Based/1(dataIn)
  Variable Delay RAM Based/1(dataOut) -> dataOut/1
  d/1 -> Variable Delay RAM Based/3(d)

== system soc_range_doppler_fpga/Radar Target Emulator/Pack Data/Pack Vector ==
  u : Inport
  pack_vector : MATLAB Function  TreatAsAtomicUnit=on
  y : Outport
  wires:
  pack_vector/1(y) -> y/1
  u/1 -> pack_vector/1(u)

== system soc_range_doppler_fpga/Radar Target Emulator/Pack Data/Pack Vector1 ==
  u : Inport
  pack_vector : MATLAB Function  TreatAsAtomicUnit=on
  y : Outport
  wires:
  u/1 -> pack_vector/1(u)
  pack_vector/1(y) -> y/1

== system soc_range_doppler_fpga/Range Doppler Tx-Rx/ADC Interface/Unpack Vector I ==
  In1 : Inport
  Data Type Conversion : DataTypeConversion  OutDataTypeStr=datatype  ConvertRealWorld=Stored Integer (SI)  SaturateOnIntegerOverflow=off  RndMeth=Floor
  MATLAB Function : MATLAB Function  TreatAsAtomicUnit=on
  Reshape : Reshape  OutputDimensionality=Column vector (2-D)
  Signal Specification : SignalSpecification  Dimensions=VectorLength
  Out1 : Outport  VectorParamsAs1DForOutWhenUnconnected=off
  wires:
  In1/1 -> MATLAB Function/1(packed_in)
  MATLAB Function/1(vec_out) -> Data Type Conversion/1
  Reshape/1 -> Out1/1
  Data Type Conversion/1 -> Signal Specification/1
  Signal Specification/1 -> Reshape/1

== system soc_range_doppler_fpga/Range Doppler Tx-Rx/ADC Interface/Unpack Vector Q ==
  In1 : Inport
  Data Type Conversion : DataTypeConversion  OutDataTypeStr=datatype  ConvertRealWorld=Stored Integer (SI)  SaturateOnIntegerOverflow=off  RndMeth=Floor
  MATLAB Function : MATLAB Function  TreatAsAtomicUnit=on
  Reshape : Reshape  OutputDimensionality=Column vector (2-D)
  Signal Specification : SignalSpecification  Dimensions=VectorLength
  Out1 : Outport  VectorParamsAs1DForOutWhenUnconnected=off
  wires:
  Signal Specification/1 -> Reshape/1
  Data Type Conversion/1 -> Signal Specification/1
  Reshape/1 -> Out1/1
  MATLAB Function/1(vec_out) -> Data Type Conversion/1
  In1/1 -> MATLAB Function/1(packed_in)

== system soc_range_doppler_fpga/Range Doppler Tx-Rx/DAC Interface/Pack Vector I ==
  u : Inport
  pack_vector : MATLAB Function  TreatAsAtomicUnit=on
  y : Outport
  wires:
  pack_vector/1(y) -> y/1
  u/1 -> pack_vector/1(u)

== system soc_range_doppler_fpga/Range Doppler Tx-Rx/DAC Interface/Pack Vector Q ==
  u : Inport
  pack_vector : MATLAB Function  TreatAsAtomicUnit=on
  y : Outport
  wires:
  u/1 -> pack_vector/1(u)
  pack_vector/1(y) -> y/1

== system soc_range_doppler_fpga/Range Doppler Tx-Rx/DMA Interface/Pack Complex Vector ==
  u : Inport
  pack_vector_complex : MATLAB Function  TreatAsAtomicUnit=on
  y : Outport
  wires:
  pack_vector_complex/1(y) -> y/1
  u/1 -> pack_vector_complex/1(u)

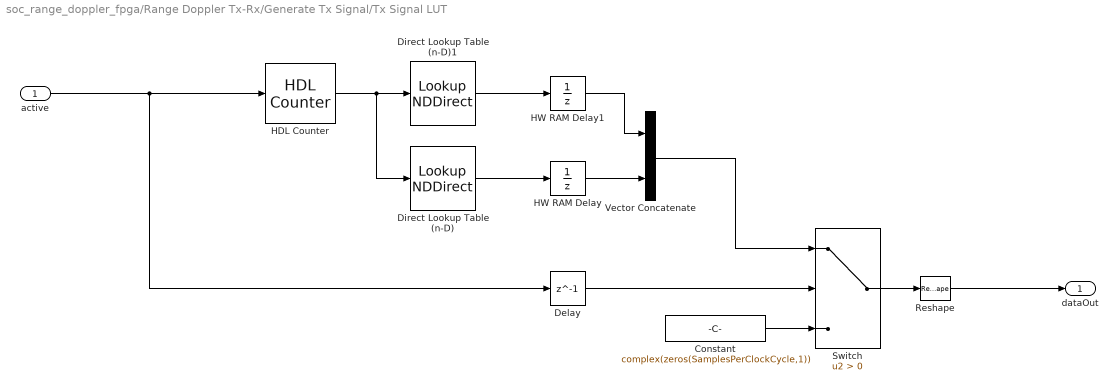
== system soc_range_doppler_fpga/Range Doppler Tx-Rx/Generate Tx Signal/Tx Signal LUT ==
  active : Inport
  Constant : Constant  Value=complex(zeros(SamplesPerClockCycle,1))  OutDataTypeStr=Inherit: Inherit via back propagation  SampleTime=-1
  Delay : Delay  DelayLength=1
  Direct Lookup Table (n-D) : LookupNDDirect  NumberOfTableDimensions=1  Table=txSignal(2:2:end)  DiagnosticForOutOfRangeInput=Error  TableDataTypeStr=outputDT
  Direct Lookup Table (n-D)1 : LookupNDDirect  NumberOfTableDimensions=1  Table=txSignal(1:2:end)  DiagnosticForOutOfRangeInput=Error  TableDataTypeStr=outputDT
  HDL Counter : hdlsllib/Sources/HDL Counter  CountType=Free running  CountInit=0  CountStep=1  CountMax=25  CountFromType=Initial value  CountFrom=0  CountResetPort=off  CountLoadPort=off  CountEnbPort=on  CountDirPort=off  CountHitOutputPort=off  CountDataType=Unsigned  CountWordLen=nextpow2(length(txSignal)/2)  CountFracLen=0  CountSampTime=1
  HW RAM Delay : UnitDelay  SampleTime=-1  HasFrameUpgradeWarning=on
  HW RAM Delay1 : UnitDelay  SampleTime=-1  HasFrameUpgradeWarning=on
  Reshape : Reshape  OutputDimensionality=Column vector (2-D)
  Switch : Switch  Criteria=u2 > Threshold  SaturateOnIntegerOverflow=off  InputSameDT=off
  Vector Concatenate : Concatenate
  dataOut : Outport
  wires:
  HDL Counter/1 -> Direct Lookup Table (n-D)/1, Direct Lookup Table (n-D)1/1
  Direct Lookup Table (n-D)/1 -> HW RAM Delay/1
  Direct Lookup Table (n-D)1/1 -> HW RAM Delay1/1
  HW RAM Delay/1 -> Vector Concatenate/2
  HW RAM Delay1/1 -> Vector Concatenate/1
  active/1 -> HDL Counter/1, Delay/1
  Constant/1 -> Switch/3
  Vector Concatenate/1 -> Switch/1
  Switch/1 -> Reshape/1
  Delay/1 -> Switch/2
  Reshape/1 -> dataOut/1

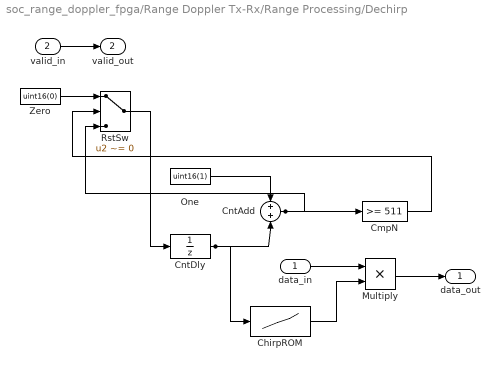
== system soc_range_doppler_fpga/Range Doppler Tx-Rx/Range Processing/Dechirp ==
  data_in : Inport
  valid_in : Inport  Port=2
  ChirpROM : Lookup_n-D  NumberOfTableDimensions=1  BreakpointsForDimension1=[0 1 2 3 4 5 6 7 8 9 10 11 12 13 14 15 16 17 18 19 20 21 22 23 24 25 26 27 28 29 30 31 32 33 34 35 36 37 38 39 40 41 42 43 44 45 46 47 48 49 50 51 52 53 54 55 56 57 58 59 60 61 62 63 64 65 66 67 68 69 70 71 72 73 74 75 76 77 78 79 80 81 82 83 84 85 86 87 88 89 90 91 92 93 94 95 96 97 98 99 100 101 102 103 104 105 106 107 108 109 110 111 112 113 114 115 116 117 118 119 120 121 122 123 124 125 126 127 128 129 130 131 132 133 134 135 136 137 138 139 140 141 142 143 144 145 146 147 148 149 150 151 152 153 154 155 156 157 158 159 160 161 162 163 164 165 166 167 168 169 170 171 172 173 174 175 176 177 178 179 180 181 182 183 184 185 186 187 188 189 190 191 192 193 194 195 196 197 198 199 200 201 202 203 204 205 206 207 208 209 210 211 212 213 214 215 216 217 218 219 220 221 222 223 224 225 226 227 228 229 230 231 232 233 234 235 236 237 238 239 240 241 242 243 244 245 246 247 248 249 250 251 252 253 254 255 256 257 258 259 260 261 262 263 264 265 266 267 268 269 270 271 272 273 274 275 276 277 278 279 280 281 282 283 284 285 286 287 288 289 290 291 292 293 294 295 296 297 298 299 300 301 302 303 304 305 306 307 308 309 310 311 312 313 314 315 316 317 318 319 320 321 322 323 324 325 326 327 328 329 330 331 332 333 334 335 336 337 338 339 340 341 342 343 344 345 346 347 348 349 350 351 352 353 354 355 356 357 358 359 360 361 362 363 364 365 366 367 368 369 370 371 372 373 374 375 376 377 378 379 380 381 382 383 384 385 386 387 388 389 390 391 392 393 394 395 396 397 398 399 400 401 402 403 404 405 406 407 408 409 410 411 412 413 414 415 416 417 418 419 420 421 422 423 424 425 426 427 428 429 430 431 432 433 434 435 436 437 438 439 440 441 442 443 444 445 446 447 448 449 450 451 452 453 454 455 456 457 458 459 460 461 462 463 464 465 466 467 468 469 470 471 472 473 474 475 476 477 478 479 480 481 482 483 484 485 486 487 488 489 490 491 492 493 494 495 496 497 498 499 500 501 502 503 504 505 506 507 508 509 510 511]  Table=[1;0.999973;0.999566;0.997805;0.993068;0.983105;0.965074;0.935617;0.891007;0.827356;0.740951;0.628684;0.488621;0.320665;0.127281;-0.0857973;-0.309017;-0.528762;-0.727623;-0.885368;-0.980785;-0.994436;-0.91221;-0.729305;-0.45399;-0.110222;0.261979;0.60941;0.872496;0.995879;0.941544;0.701881;0.309017;-0.163703;-0.611354;-0.919114;-0.993068;-0.792855;-0.355311;0.202307;0.707107;0.982195;0.91221;0.499291;-0.117537;-0.698376;-0.991867;-0.84877;-0.309017;0.389476;0.903989;0.954777;0.488621;-0.259609;-0.867657;-0.960431;-0.45399;0.353016;0.934748;0.878426;0.19509;-0.640068;-0.999566;-0.581812;0.309017;0.953306;0.791357;-0.0662195;-0.872496;-0.878426;-0.0490677;0.835538;0.891007;0.0319014;-0.867657;-0.838225;0.117537;0.947193;0.685977;-0.389476;-1;-0.37587;0.727623;0.896511;-0.117537;-0.978317;-0.497163;0.684189;0.891007;-0.202307;-0.998795;-0.283231;0.872496;0.65873;-0.611354;-0.88764;0.309017;0.98651;-0.0294482;-0.995879;-0.19509;0.959052;0.355311;-0.911201;-0.45399;0.87607;0.497163;-0.866434;-0.488621;0.885368;0.427555;-0.926672;-0.309017;0.974062;0.127281;-0.999925;0.117537;0.965714;-0.409724;-0.827356;0.707107;0.549433;-0.934748;-0.129715;0.993068;-0.371317;-0.791357;0.813323;0.309017;-0.999973;0.33689;0.768318;-0.872496;-0.129715;0.965074;-0.624859;-0.45399;0.999491;-0.409724;-0.628684;0.980785;-0.297323;-0.685977;0.974062;-0.309017;-0.643832;0.991867;-0.443022;-0.488621;0.994436;-0.671559;-0.187863;0.891007;-0.911201;0.261979;0.565732;-0.993068;0.752379;-0.0294482;-0.701881;1;-0.712294;0.0294482;0.65873;-0.993068;0.824589;-0.261979;-0.411962;0.891007;-0.982195;0.671559;-0.105342;-0.488621;0.896511;-0.991867;0.765167;-0.309017;-0.226279;0.685977;-0.954777;0.980785;-0.777661;0.409724;0.0319014;-0.45399;0.780737;-0.965074;0.991551;-0.872496;0.640068;-0.33689;0.00736304;0.309017;-0.581812;0.791357;-0.928506;0.993068;-0.991551;0.934748;-0.835538;0.707107;-0.561677;0.409724;-0.259609;0.117537;0.0122715;-0.127281;0.226279;-0.309017;0.37587;-0.427555;0.46489;-0.488621;0.499291;-0.497163;0.482184;-0.45399;0.411962;-0.355311;0.283231;-0.19509;0.0906869;0.0294482;-0.163703;0.309017;-0.460539;0.611354;-0.752379;0.872496;-0.959052;0.998795;-0.979322;0.891007;-0.729305;0.497163;-0.207111;-0.117537;0.443022;-0.727623;0.926672;-1;0.921037;-0.685977;0.320665;0.117537;-0.545325;0.867657;-0.999491;0.891007;-0.549433;0.0490677;0.477878;-0.872496;0.997805;-0.791357;0.302006;0.309017;-0.813323;0.999566;-0.768318;0.19509;0.477878;-0.934748;0.935617;-0.45399;-0.27852;0.867657;-0.965714;0.488621;0.297323;-0.903989;0.921037;-0.309017;-0.528762;0.991867;-0.715731;-0.117537;0.866434;-0.91221;0.187863;0.707107;-0.979322;0.355311;0.60941;-0.993068;0.393992;0.611354;-0.98651;0.309017;0.712294;-0.941544;0.0906869;0.872496;-0.792855;-0.261979;0.993907;-0.45399;-0.684189;0.91221;0.105342;-0.980785;0.46489;0.727623;-0.84877;-0.309017;0.996313;-0.127281;-0.947193;0.488621;0.777661;-0.740951;-0.561677;0.891007;0.353016;-0.965074;-0.18304;0.993068;0.0662195;-0.999566;-0.00736304;1;0.00736304;-0.999566;-0.0662195;0.993068;0.18304;-0.965074;-0.353016;0.891007;0.561677;-0.740951;-0.777661;0.488621;0.947193;-0.127281;-0.996313;-0.309017;0.84877;0.727623;-0.46489;-0.980785;-0.105342;0.91221;0.684189;-0.45399;-0.993907;-0.261979;0.792855;0.872496;-0.0906869;-0.941544;-0.712294;0.309017;0.98651;0.611354;-0.393992;-0.993068;-0.60941;0.355311;0.979322;0.707107;-0.187863;-0.91221;-0.866434;-0.117537;0.715731;0.991867;0.528762;-0.309017;-0.921037;-0.903989;-0.297323;0.488621;0.965714;0.867657;0.27852;-0.45399;-0.935617;-0.934748;-0.477878;0.19509;0.768318;0.999566;0.813323;0.309017;-0.302006;-0.791357;-0.997805;-0.872496;-0.477878;0.0490677;0.549433;0.891007;0.999491;0.867657;0.545325;0.117537;-0.320665;-0.685977;-0.921037;-1;-0.926672;-0.727623;-0.443022;-0.117537;0.207111;0.497163;0.729305;0.891007;0.979322;0.998795;0.959052;0.872496;0.752379;0.611354;0.460539;0.309017;0.163703;0.0294482;-0.0906869;-0.19509;-0.283231;-0.355311;-0.411962;-0.45399;-0.482184;-0.497163 ...(+799 chars)]  InterpMethod=Flat  InternalRulePriority=Speed  OutDataTypeStr=filterOutDT  RndMeth=Simplest
  CmpN : simulink/Logic and Bit Operations/Compare To Constant  relop=>=  const=511  OutDataTypeStr=boolean
  CntAdd : Sum  OutDataTypeStr=uint16
  CntDly : UnitDelay  SampleTime=8e-09  HasFrameUpgradeWarning=on
  Multiply : Product  OutDataTypeStr=filterOutDT
  One : Constant  Value=uint16(1)  OutDataTypeStr=uint16
  RstSw : Switch  Criteria=u2 ~= 0  SaturateOnIntegerOverflow=off  InputSameDT=off
  Zero : Constant  Value=uint16(0)  OutDataTypeStr=uint16
  data_out : Outport
  valid_out : Outport  Port=2
  wires:
  valid_in/1 -> valid_out/1
  ChirpROM/1 -> Multiply/2
  RstSw/1 -> CntDly/1
  data_in/1 -> Multiply/1
  Zero/1 -> RstSw/1
  One/1 -> CntAdd/1
  CntAdd/1 -> RstSw/3, CmpN/1
  CntDly/1 -> CntAdd/2, ChirpROM/1
  CmpN/1 -> RstSw/2
  Multiply/1 -> data_out/1

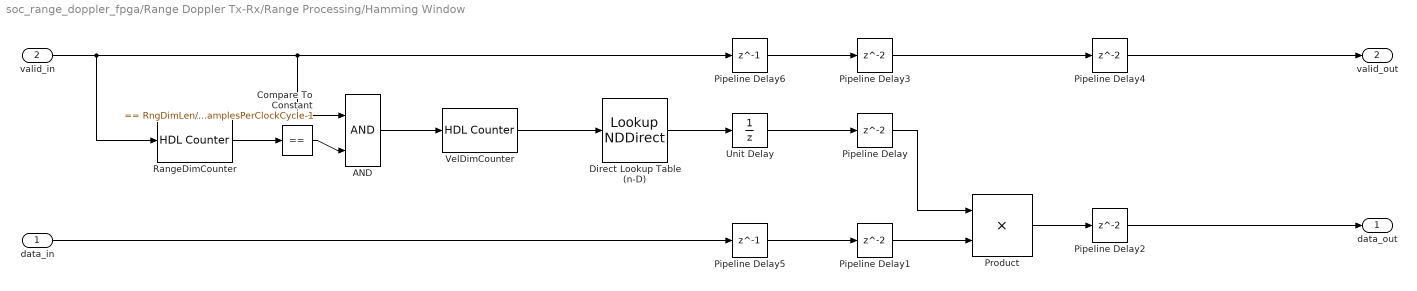
== system soc_range_doppler_fpga/Range Doppler Tx-Rx/Range Processing/Hamming Window ==
  data_in : Inport
  valid_in : Inport  Port=2
  AND : Logic  IconShape=distinctive  AllPortsSameDT=off  OutDataTypeStr=boolean
  Compare To Constant : simulink/Logic and Bit Operations/Compare To Constant  relop===  const=RngDimLen/SamplesPerClockCycle-1  OutDataTypeStr=boolean
  Direct Lookup Table (n-D) : LookupNDDirect  NumberOfTableDimensions=1  Table=hamming(VelDimLen)  DiagnosticForOutOfRangeInput=Error  TableDataTypeStr=fixdt(1,18,16)
  Pipeline Delay{,1..4} (5 alike) : Delay
  Pipeline Delay5 : Delay  DelayLength=1
  Pipeline Delay6 : Delay  DelayLength=1
  Product : Product
  RangeDimCounter : hdlsllib/Sources/HDL Counter  CountType=Free running  CountInit=0  CountStep=1  CountMax=25  CountFromType=Initial value  CountFrom=0  CountResetPort=off  CountLoadPort=off  CountEnbPort=on  CountDirPort=off  CountHitOutputPort=off  CountDataType=Unsigned  CountWordLen=nextpow2(RngDimLen/SamplesPerClockCycle)  CountFracLen=0  CountSampTime=1
  Unit Delay : UnitDelay  SampleTime=-1  HasFrameUpgradeWarning=on
  VelDimCounter : hdlsllib/Sources/HDL Counter  CountType=Free running  CountInit=0  CountStep=1  CountMax=25  CountFromType=Initial value  CountFrom=0  CountResetPort=off  CountLoadPort=off  CountEnbPort=on  CountDirPort=off  CountHitOutputPort=off  CountDataType=Unsigned  CountWordLen=nextpow2(VelDimLen)  CountFracLen=0  CountSampTime=1
  data_out : Outport  VectorParamsAs1DForOutWhenUnconnected=off
  valid_out : Outport  Port=2  VectorParamsAs1DForOutWhenUnconnected=off
  wires:
  Product/1 -> Pipeline Delay2/1
  data_in/1 -> Pipeline Delay5/1
  Pipeline Delay/1 -> Product/1
  Pipeline Delay1/1 -> Product/2
  valid_in/1 -> RangeDimCounter/1, Pipeline Delay6/1, AND/1
  Pipeline Delay3/1 -> Pipeline Delay4/1
  Pipeline Delay4/1 -> valid_out/1
  Pipeline Delay2/1 -> data_out/1
  Unit Delay/1 -> Pipeline Delay/1
  Pipeline Delay5/1 -> Pipeline Delay1/1
  Pipeline Delay6/1 -> Pipeline Delay3/1
  Direct Lookup Table (n-D)/1 -> Unit Delay/1
  VelDimCounter/1 -> Direct Lookup Table (n-D)/1
  RangeDimCounter/1 -> Compare To Constant/1
  Compare To Constant/1 -> AND/2
  AND/1 -> VelDimCounter/1

== system soc_range_doppler_fpga/Radar Target Emulator/Multiple Target Emulator/Unpack Data/Unpack Vector ==
  In1 : Inport
  Data Type Conversion : DataTypeConversion  OutDataTypeStr=datatype  ConvertRealWorld=Stored Integer (SI)  SaturateOnIntegerOverflow=off  RndMeth=Floor
  MATLAB Function : MATLAB Function  TreatAsAtomicUnit=on
  Reshape : Reshape  OutputDimensionality=Column vector (2-D)
  Out1 : Outport  VectorParamsAs1DForOutWhenUnconnected=off
  wires:
  Data Type Conversion/1 -> Reshape/1
  In1/1 -> MATLAB Function/1(packed_in)
  MATLAB Function/1(vec_out) -> Data Type Conversion/1
  Reshape/1 -> Out1/1

== system soc_range_doppler_fpga/Radar Target Emulator/Multiple Target Emulator/Unpack Data/Unpack Vector1 ==
  In1 : Inport
  Data Type Conversion : DataTypeConversion  OutDataTypeStr=datatype  ConvertRealWorld=Stored Integer (SI)  SaturateOnIntegerOverflow=off  RndMeth=Floor
  MATLAB Function : MATLAB Function  TreatAsAtomicUnit=on
  Reshape : Reshape  OutputDimensionality=Column vector (2-D)
  Out1 : Outport  VectorParamsAs1DForOutWhenUnconnected=off
  wires:
  Reshape/1 -> Out1/1
  MATLAB Function/1(vec_out) -> Data Type Conversion/1
  In1/1 -> MATLAB Function/1(packed_in)
  Data Type Conversion/1 -> Reshape/1

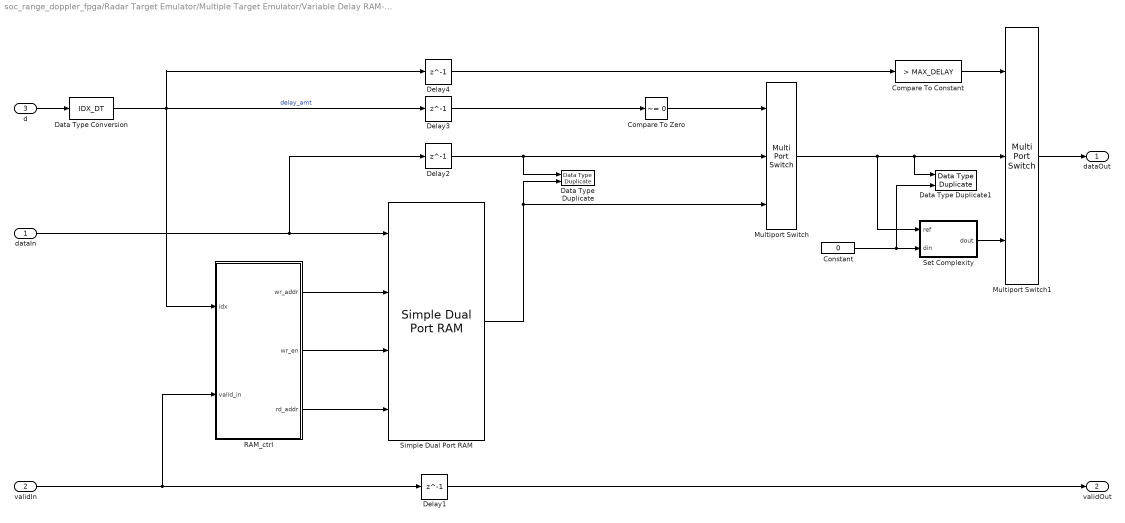
== system soc_range_doppler_fpga/Radar Target Emulator/Multiple Target Emulator/Variable Delay RAM-based/Variable Delay RAM Based ==
  dataIn : Inport
  validIn : Inport  Port=2  OutDataTypeStr=boolean
  d : Inport  Port=3
  Compare To Constant : simulink/Logic and Bit Operations/Compare To Constant  relop=>  const=MAX_DELAY  OutDataTypeStr=boolean
  Compare To Zero : simulink/Logic and Bit Operations/Compare To Zero  relop=~=  OutDataTypeStr=boolean
  Constant : Constant  Value=0  OutDataTypeStr=Inherit: Inherit via back propagation  SampleTime=-1
  Data Type Duplicate : DataTypeDuplicate
  Data Type Duplicate1 : DataTypeDuplicate
  Data Type Conversion : DataTypeConversion  OutDataTypeStr=IDX_DT  SaturateOnIntegerOverflow=off  RndMeth=Floor
  Delay{1..4} (4 alike) : Delay  DelayLength=1
  Multiport Switch : MultiPortSwitch  DataPortOrder=Zero-based contiguous  Inputs=2  zeroidx=on  SaturateOnIntegerOverflow=off  InputSameDT=off
  Multiport Switch1 : MultiPortSwitch  DataPortOrder=Zero-based contiguous  Inputs=2  zeroidx=on  SaturateOnIntegerOverflow=off  InputSameDT=off
  RAM_ctrl : Subsystem
  Set Complexity : MATLAB Function  TreatAsAtomicUnit=on
  Simple Dual Port RAM : hdlsllib/HDL RAMs/Simple Dual Port RAM  ram_size=ADDR_WIDTH
  dataOut : Outport  VectorParamsAs1DForOutWhenUnconnected=off
  validOut : Outport  Port=2  VectorParamsAs1DForOutWhenUnconnected=off
  wires:
  RAM_ctrl/2(wr_en) -> Simple Dual Port RAM/3
  RAM_ctrl/1(wr_addr) -> Simple Dual Port RAM/2
  d/1 -> Data Type Conversion/1
  Simple Dual Port RAM/1 -> Data Type Duplicate/2, Multiport Switch/3
  dataIn/1 -> Simple Dual Port RAM/1, Delay2/1
  Data Type Conversion/1 -> Delay4/1, Delay3/1, RAM_ctrl/1(idx)  "delay_amt"
  Multiport Switch/1 -> Set Complexity/1(ref), Data Type Duplicate1/1, Multiport Switch1/2
  Multiport Switch1/1 -> dataOut/1
  Compare To Constant/1 -> Multiport Switch1/1
  Delay1/1 -> validOut/1
  Delay2/1 -> Data Type Duplicate/1, Multiport Switch/2
  RAM_ctrl/3(rd_addr) -> Simple Dual Port RAM/4
  validIn/1 -> Delay1/1, RAM_ctrl/2(valid_in)
  Compare To Zero/1 -> Multiport Switch/1
  Delay3/1 -> Compare To Zero/1
  Delay4/1 -> Compare To Constant/1
  Set Complexity/1(dout) -> Multiport Switch1/3
  Constant/1 -> Set Complexity/2(din), Data Type Duplicate1/2
